simulink model "power_transformer"  (Simulink 6.0)
settings: Solver=ode15s  SolverMode=SingleTasking  StartTime=0.0  StopTime=0.1  RelTol=1e-3  AbsTol=1e-6
libraries: powerlib x11
settings Model: Creator=patrice  LastModifiedBy=batserve  ExtModeTrigMode=oneshot  ExtModeArmWhenConnect=off  ExtModeAutoUpdateStatusClock=off
settings DataIOCC: LimitDataPoints=off  SignalLoggingName=sigsOut
settings OptimizationCC: BooleanDataType=off
settings DebuggingCC: SolverPrmCheckMsg=none
settings HardwareCC: TargetUnknown=on
settings RTWCC: TemplateMakefile=grt_unix.tmf

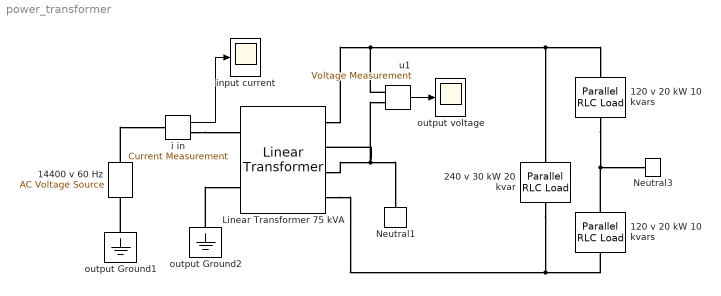
== system power_transformer ==
  120 v 20 kW 10 kvars : powerlib/Elements/Parallel RLC Load  Orientation=down  PhysicalDomain=powersysdomain  SubClassName=unknown  PortType=p1  LConnTagsString=a  RConnTagsString=__new0  NominalVoltage=120  NominalFrequency=60  ActivePower=20e3  InductivePower=10e3  CapacitivePower=0  Measurements=None
      settings: AttributesFormatString=\n
  "120 v 20 kW 10 kvars " : powerlib/Elements/Parallel RLC Load  Orientation=up  PhysicalDomain=powersysdomain  SubClassName=unknown  PortType=p1  LConnTagsString=a  RConnTagsString=__new0  NominalVoltage=120  NominalFrequency=60  ActivePower=20e3  InductivePower=10e3  CapacitivePower=0  Measurements=None
      settings: AttributesFormatString=\n
  14400 v 60 Hz : powerlib/Electrical Sources/AC Voltage Source  Description=source block  Orientation=up  Amplitude=14400*sqrt(2)  Phase=0  Frequency=60  SampleTime=0  Measurements=None
      settings: AttributesFormatString=\n
  240 v 30 kW 20 kvar : powerlib/Elements/Parallel RLC Load  Orientation=down  PhysicalDomain=powersysdomain  SubClassName=unknown  PortType=p1  LConnTagsString=a  RConnTagsString=__new0  NominalVoltage=240  NominalFrequency=60  ActivePower=30e3  InductivePower=0  CapacitivePower=20e3  Measurements=None
      settings: AttributesFormatString=\n
  "Linear Transformer 75 kVA " : powerlib/Elements/Linear Transformer  PhysicalDomain=powersysdomain  SubClassName=unknown  PortType=p1  LConnTagsString=a|b  RConnTagsString=A|B|C|D  NominalPower=[75e3,60]  winding1=[14.4e3 0.01,0.03]  winding2=[120,0.02,0]  ThreeWindings=on  winding3=[120,0.02,0]  RmLm=[50,50]  Measurements=None
  Neutral1 : powerlib/Elements/Neutral  Orientation=down  PhysicalDomain=powersysdomain  SubClassName=unknown  PortType=p1  LConnTagsString=a  NodeNumber=50
  Neutral3 : powerlib/Elements/Neutral  PhysicalDomain=powersysdomain  SubClassName=unknown  PortType=p1  LConnTagsString=a  NodeNumber=50
  i in : powerlib/Measurements/Current Measurement  Tag=PoWeRsYsTeMmEaSuReMeNt  PhasorSimulation=off  OutputType=Magnitude  PSBequivalent=0
  input current : Scope
      settings: DeleteFcn=simscope BlockIsBeingDestroyed  PostSaveFcn=simscope Save  TickLabels=on  TimeRange=0.1  YMin=-10  YMax=10  DataFormat=Array
  output voltage : Scope
      settings: DeleteFcn=simscope BlockIsBeingDestroyed  PostSaveFcn=simscope Save  TickLabels=on  TimeRange=0.1  YMin=-200  YMax=200  DataFormat=Array
  output Ground1 : powerlib/Elements/Ground  Orientation=down  PhysicalDomain=powersysdomain  SubClassName=unknown  PortType=p1  LConnTagsString=a
  output Ground2 : powerlib/Elements/Ground  Orientation=down  PhysicalDomain=powersysdomain  SubClassName=unknown  PortType=p1  LConnTagsString=a
  u1 : powerlib/Measurements/Voltage Measurement  Tag=PoWeRsYsTeMmEaSuReMeNt  PhasorSimulation=off  OutputType=Magnitude  PSBequivalent=0
  wires:
  i in/1 -> input current/1
  u1/1 -> output voltage/1
  connections:
  output Ground2/LConn1 -- "Linear Transformer 75 kVA "/LConn2
  output Ground1/LConn1 -- 14400 v 60 Hz/LConn1
  "120 v 20 kW 10 kvars "/RConn1 -- Neutral3/LConn1 -- 120 v 20 kW 10 kvars/RConn1
  14400 v 60 Hz/RConn1 -- i in/LConn1
  i in/RConn1 -- "Linear Transformer 75 kVA "/LConn1
  "Linear Transformer 75 kVA "/RConn3 -- "Linear Transformer 75 kVA "/RConn2 -- Neutral1/LConn1 -- u1/LConn2
  u1/LConn1 -- 240 v 30 kW 20 kvar/LConn1 -- 120 v 20 kW 10 kvars/LConn1 -- "Linear Transformer 75 kVA "/RConn1
  "Linear Transformer 75 kVA "/RConn4 -- "120 v 20 kW 10 kvars "/LConn1 -- 240 v 30 kW 20 kvar/RConn1
